simulink model "NeuroControl_Loudspeaker_offline2"  (R2016a)
settings: Solver=ode5  StartTime=0.0  StopTime=0.1  FixedStep=1/fs  RelTol=1e-3
values from neighbouring files (symbols this model uses):
  AaLinear = [0,1,0,0; -(K)/Md,-Rmd/Md,0,A/Md; 0,0,0,1; 0,-A/(L0+Ld),-(1/Cd)/(L0+Ld),-(Re0+Red)/(L0+Ld)]    [NeuroControl_loudspeaker.m]    (also in NeuroControl_loudspeaker2.m; NeuroControl_loudspeaker_LinearPlusNN.m; NeuroControl_loudspeaker_MoreLikeMachineLearning.m; NeuroControl_loudspeaker_MoreLikeMachineLearning_deep.m)
  Anlr = zeros(4,4)    [NeuroControl_loudspeaker.m]    (also in NeuroControl_loudspeaker2.m; NeuroControl_loudspeaker_LinearPlusNN.m; NeuroControl_loudspeaker_MoreLikeMachineLearning.m; NeuroControl_loudspeaker_MoreLikeMachineLearning_deep.m)
  Anlr2 = zeros(4,4)    [NeuroControl_loudspeaker.m]    (also in NeuroControl_loudspeaker2.m; NeuroControl_loudspeaker_LinearPlusNN.m; NeuroControl_loudspeaker_MoreLikeMachineLearning.m; NeuroControl_loudspeaker_MoreLikeMachineLearning_deep.m)
  Anlr3 = zeros(4,4)    [NeuroControl_loudspeaker.m]    (also in NeuroControl_loudspeaker2.m; NeuroControl_loudspeaker_LinearPlusNN.m; NeuroControl_loudspeaker_MoreLikeMachineLearning.m; NeuroControl_loudspeaker_MoreLikeMachineLearning_deep.m)
  Atemp = A    (= 5.62)    [NeuroControl_loudspeaker.m]    (also in NeuroControl_loudspeaker2.m; NeuroControl_loudspeaker_LinearPlusNN.m; NeuroControl_loudspeaker_MoreLikeMachineLearning.m; NeuroControl_loudspeaker_MoreLikeMachineLearning_deep.m)
  Ba = [0,0,0,1/(L0+Ld)]'    [NeuroControl_loudspeaker.m]    (also in NeuroControl_loudspeaker2.m; NeuroControl_loudspeaker_LinearPlusNN.m; NeuroControl_loudspeaker_MoreLikeMachineLearning.m; NeuroControl_loudspeaker_MoreLikeMachineLearning_deep.m)
  fInput = 60    [NeuroControl_loudspeaker.m]    (also in NeuroControl_loudspeaker2.m; NeuroControl_loudspeaker_LinearPlusNN.m; NeuroControl_loudspeaker_MoreLikeMachineLearning.m; NeuroControl_loudspeaker_MoreLikeMachineLearning_deep.m)
  fs = fs/downrate    (= 48000)    [NeuroControl_loudspeaker.m]    (also in NeuroControl_loudspeaker2.m; NeuroControl_loudspeaker_LinearPlusNN.m; NeuroControl_loudspeaker_MoreLikeMachineLearning.m; NeuroControl_loudspeaker_MoreLikeMachineLearning_deep.m)
  fsSim = 48000    [NeuroControl_loudspeaker.m]    (also in NeuroControl_loudspeaker2.m; NeuroControl_loudspeaker_LinearPlusNN.m; NeuroControl_loudspeaker_MoreLikeMachineLearning.m; NeuroControl_loudspeaker_MoreLikeMachineLearning_deep.m)
  G = Gt'    [NeuroControl_loudspeaker.m]    (also in NeuroControl_loudspeaker2.m; NeuroControl_loudspeaker_LinearPlusNN.m; NeuroControl_loudspeaker_MoreLikeMachineLearning.m; NeuroControl_loudspeaker_MoreLikeMachineLearning_deep.m)
  gain = 1/zpkerasys(1,1).k    [NeuroControl_loudspeaker.m]    (also in NeuroControl_loudspeaker2.m; NeuroControl_loudspeaker_LinearPlusNN.m; NeuroControl_loudspeaker_MoreLikeMachineLearning.m; NeuroControl_loudspeaker_MoreLikeMachineLearning_deep.m)
  InputGain = 1    [NeuroControl_loudspeaker.m]    (also in NeuroControl_loudspeaker2.m; NeuroControl_loudspeaker_LinearPlusNN.m; NeuroControl_loudspeaker_MoreLikeMachineLearning.m; NeuroControl_loudspeaker_MoreLikeMachineLearning_deep.m)
  inputGainForPushingNonlinearity = 5    [NeuroControl_loudspeaker.m]    (also in NeuroControl_loudspeaker2.m; NeuroControl_loudspeaker_LinearPlusNN.m = 10; NeuroControl_loudspeaker_MoreLikeMachineLearning.m = 10; NeuroControl_loudspeaker_MoreLikeMachineLearning_deep.m = 10)
  inverseFilterGainCompensation = 1/0.0054    (= 185.185185185)    [NeuroControl_loudspeaker.m]    (also in NeuroControl_loudspeaker2.m; NeuroControl_loudspeaker_LinearPlusNN.m; NeuroControl_loudspeaker_MoreLikeMachineLearning.m; NeuroControl_loudspeaker_MoreLikeMachineLearning_deep.m)
  K = Kd    (= 4538)    [NeuroControl_loudspeaker.m]    (also in NeuroControl_loudspeaker2.m; NeuroControl_loudspeaker_LinearPlusNN.m; NeuroControl_loudspeaker_MoreLikeMachineLearning.m; NeuroControl_loudspeaker_MoreLikeMachineLearning_deep.m)
  noise = 0    [NeuroControl_loudspeaker.m]    (also in NeuroControl_loudspeaker2.m; NeuroControl_loudspeaker_LinearPlusNN.m; NeuroControl_loudspeaker_MoreLikeMachineLearning.m; NeuroControl_loudspeaker_MoreLikeMachineLearning_deep.m)
  ObserverNorm = 1    [NeuroControl_loudspeaker.m]    (also in NeuroControl_loudspeaker2.m; NeuroControl_loudspeaker_LinearPlusNN.m; NeuroControl_loudspeaker_MoreLikeMachineLearning.m; NeuroControl_loudspeaker_MoreLikeMachineLearning_deep.m)
  pole = z_svd    [NeuroControl_loudspeaker.m]    (also in NeuroControl_loudspeaker2.m; NeuroControl_loudspeaker_LinearPlusNN.m; NeuroControl_loudspeaker_MoreLikeMachineLearning.m; NeuroControl_loudspeaker_MoreLikeMachineLearning_deep.m)
  Rmd = 2.34    [NeuroControl_loudspeaker.m]    (also in NeuroControl_loudspeaker2.m; NeuroControl_loudspeaker_LinearPlusNN.m; NeuroControl_loudspeaker_MoreLikeMachineLearning.m; NeuroControl_loudspeaker_MoreLikeMachineLearning_deep.m)
  SignalChange = temp    (= 0)    [NeuroControl_loudspeaker.m]    (also in NeuroControl_loudspeaker2.m; NeuroControl_loudspeaker_LinearPlusNN.m; NeuroControl_loudspeaker_MoreLikeMachineLearning.m; NeuroControl_loudspeaker_MoreLikeMachineLearning_deep.m)
  sys_era_c = d2c(sys_era,'zoh')    [NeuroControl_loudspeaker.m]    (also in NeuroControl_loudspeaker2.m; NeuroControl_loudspeaker_LinearPlusNN.m; NeuroControl_loudspeaker_MoreLikeMachineLearning.m; NeuroControl_loudspeaker_MoreLikeMachineLearning_deep.m)
  zero = zpkerasys(1,1).p{1,1}    [NeuroControl_loudspeaker.m]    (also in NeuroControl_loudspeaker2.m; NeuroControl_loudspeaker_LinearPlusNN.m; NeuroControl_loudspeaker_MoreLikeMachineLearning.m; NeuroControl_loudspeaker_MoreLikeMachineLearning_deep.m)
undefined symbols (not defined in the file or in its folder): a, b
libraries: simulink x1
settings Model: Creator=kadowaki  LastModifiedBy=kadowaki
settings DataIOCC: InspectSignalLogs=on

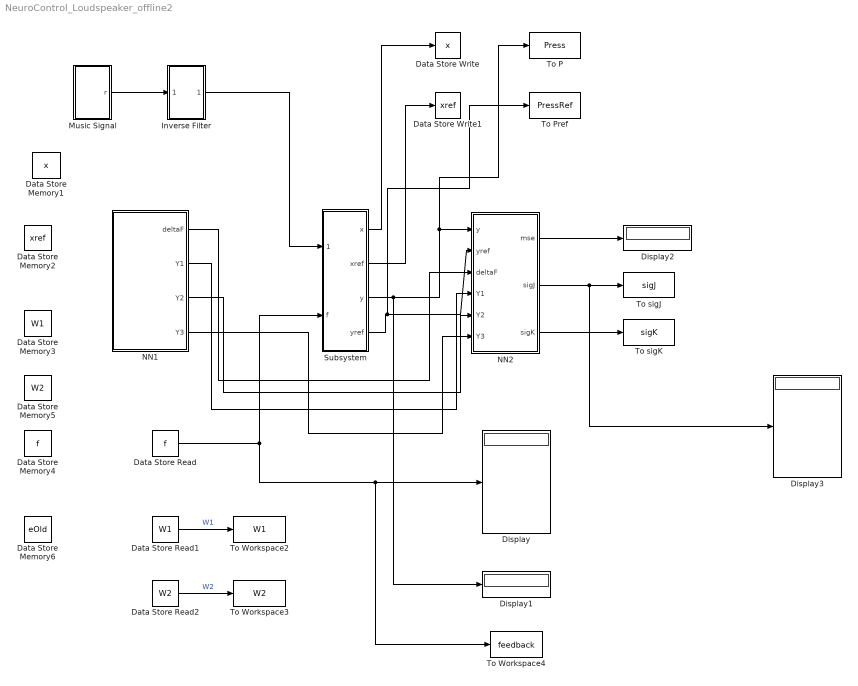
== system NeuroControl_Loudspeaker_offline2 ==
  Data Store Memory1 : DataStoreMemory  DataStoreName=x  ReadBeforeWriteMsg=warning  WriteAfterWriteMsg=warning  WriteAfterReadMsg=warning  InitialValue=zeros(6,1)  ShowAdditionalParam=off  OutDataTypeStr=double
  Data Store Memory2 : DataStoreMemory  DataStoreName=xref  ReadBeforeWriteMsg=warning  WriteAfterWriteMsg=warning  WriteAfterReadMsg=warning  InitialValue=zeros(6,1)  ShowAdditionalParam=off  OutDataTypeStr=double
  Data Store Memory3 : DataStoreMemory  DataStoreName=W1  ReadBeforeWriteMsg=warning  WriteAfterWriteMsg=warning  WriteAfterReadMsg=warning  InitialValue=W1initial  ShowAdditionalParam=off  OutDataTypeStr=double
  Data Store Memory4 : DataStoreMemory  DataStoreName=f  ReadBeforeWriteMsg=warning  WriteAfterWriteMsg=warning  WriteAfterReadMsg=warning  InitialValue=zeros(6,1)  ShowAdditionalParam=off  OutDataTypeStr=double
  Data Store Memory5 : DataStoreMemory  DataStoreName=W2  ReadBeforeWriteMsg=warning  WriteAfterWriteMsg=warning  WriteAfterReadMsg=warning  InitialValue=W2initial  ShowAdditionalParam=off  OutDataTypeStr=double
  Data Store Memory6 : DataStoreMemory  DataStoreName=eOld  ReadBeforeWriteMsg=warning  WriteAfterWriteMsg=warning  WriteAfterReadMsg=warning  ShowAdditionalParam=off  OutDataTypeStr=double
  Data Store Read : DataStoreRead  DataStoreName=f
  Data Store Read1 : DataStoreRead  DataStoreName=W1
  Data Store Read2 : DataStoreRead  DataStoreName=W2
  Data Store Write : DataStoreWrite  DataStoreName=x
  Data Store Write1 : DataStoreWrite  DataStoreName=xref
  Display{,1..3} (4 alike) : Display
  Inverse Filter : Subsystem
  Music Signal : Subsystem
  NN1 : MATLAB Function  TreatAsAtomicUnit=on
      settings: MinAlgLoopOccurrences=on
  NN2 : MATLAB Function  TreatAsAtomicUnit=on
      settings: MinAlgLoopOccurrences=on
  Subsystem : Subsystem
  To P : ToWorkspace  VariableName=Press  SaveFormat=Timeseries  SampleTime=-1
  "To Pref " : ToWorkspace  VariableName=PressRef  SaveFormat=Timeseries  SampleTime=-1
  To Workspace2 : ToWorkspace  VariableName=W1  SampleTime=-1
  To Workspace3 : ToWorkspace  VariableName=W2  SampleTime=-1
  To Workspace4 : ToWorkspace  VariableName=feedback  SampleTime=-1
  To sigJ : ToWorkspace  VariableName=sigJ  SampleTime=-1
  To sigK : ToWorkspace  VariableName=sigK  SampleTime=-1
  wires:
  Subsystem/2(xref) -> Data Store Write1/1
  Subsystem/1(x) -> Data Store Write/1
  Inverse Filter/1(Out1) -> Subsystem/1(music)
  Data Store Read/1 -> To Workspace4/1, Display/1, Subsystem/2(f)
  NN1/1(deltaF) -> NN2/3(deltaF)
  Subsystem/3(y) -> NN2/1(y), To P/1, Display1/1
  Subsystem/4(yref) -> "To Pref "/1, NN2/2(yref)
  NN1/2(Y1) -> NN2/4(Y1)
  NN1/3(Y2) -> NN2/5(Y2)
  Music Signal/1(r) -> Inverse Filter/1(In1)
  NN2/1(mse) -> Display2/1
  NN1/4(Y3) -> NN2/6(Y3)
  Data Store Read1/1 -> To Workspace2/1  "W1"
  Data Store Read2/1 -> To Workspace3/1  "W2"
  NN2/2(sigJ) -> Display3/1, To sigJ/1
  NN2/3(sigK) -> To sigK/1

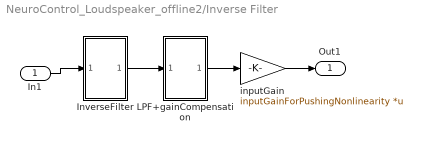
== system NeuroControl_Loudspeaker_offline2/Inverse Filter ==
  In1 : Inport
  InverseFilter : Subsystem
  LPF+gainCompensation : Subsystem
  inputGain : Gain  Gain=inputGainForPushingNonlinearity  Multiplication=Matrix(K*u)
  Out1 : Outport
  wires:
  In1/1 -> InverseFilter/1(In1)
  InverseFilter/1(Out1) -> LPF+gainCompensation/1(In1)
  LPF+gainCompensation/1(Out1) -> inputGain/1
  inputGain/1 -> Out1/1

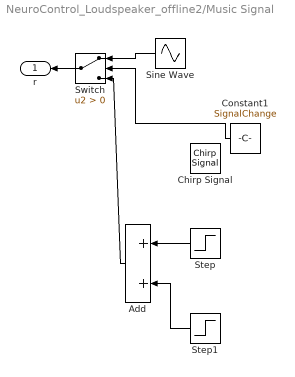
== system NeuroControl_Loudspeaker_offline2/Music Signal ==
  Add : Sum
  Chirp Signal : simulink/Sources/Chirp Signal  f1=0.1  T=2  f2=fs/2
  Constant1 : Constant  Value=SignalChange
  Sine Wave : Sin  Amplitude=InputGain  Frequency=2*pi*fInput  SampleTime=[0,0]
  Step : Step  Time=0  After=InputGain  SampleTime=[0,0]
  Step1 : Step  Time=1/fsSim  After=-InputGain  SampleTime=[0,0]
  Switch : Switch  Criteria=u2 > Threshold
  r : Outport
  wires:
  Switch/1 -> r/1
  Constant1/1 -> Switch/2
  Sine Wave/1 -> Switch/1
  Step/1 -> Add/1
  Add/1 -> Switch/3
  Step1/1 -> Add/2

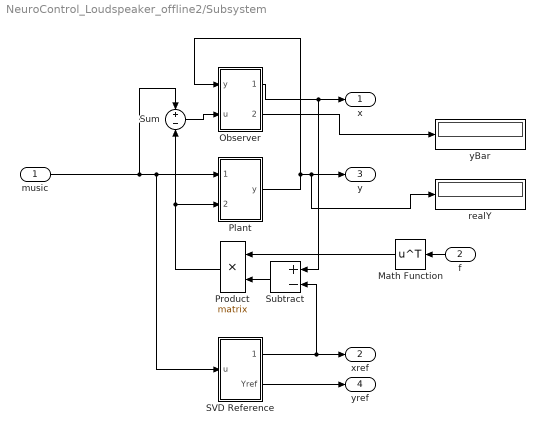
== system NeuroControl_Loudspeaker_offline2/Subsystem ==
  music : Inport
  f : Inport  Port=2
  Math Function : Math  Operator=transpose  SaturateOnIntegerOverflow=on
  Observer : Subsystem
  Plant : Subsystem
  Product : Product  Multiplication=Matrix(*)
  SVD Reference : Subsystem
  Subtract : Sum  Inputs=+-
  Sum : Sum  Inputs=+-
  realY : Display
  yBar : Display
  x : Outport
  xref : Outport  Port=2
  y : Outport  Port=3
  yref : Outport  Port=4
  wires:
  Plant/1(y) -> realY/1, y/1, Observer/1(y)
  music/1 -> Sum/1, SVD Reference/1(u), Plant/1(music)
  SVD Reference/1(Xref) -> Subtract/2, xref/1
  Observer/1(xBar) -> Subtract/1, x/1
  SVD Reference/2(Yref) -> yref/1
  f/1 -> Math Function/1
  Math Function/1 -> Product/1
  Subtract/1 -> Product/2
  Observer/2(yBar) -> yBar/1
  Product/1 -> Sum/2, Plant/2(control)
  Sum/1 -> Observer/2(u)

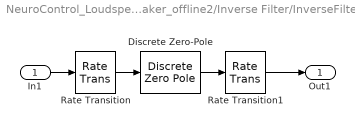
== system NeuroControl_Loudspeaker_offline2/Inverse Filter/InverseFilter ==
  In1 : Inport
  Discrete Zero-Pole : DiscreteZeroPole  Zeros=zero  Poles=pole  Gain=gain  SampleTime=1/fs
  Rate Transition : RateTransition
  Rate Transition1 : RateTransition
  Out1 : Outport
  wires:
  Rate Transition/1 -> Discrete Zero-Pole/1
  Discrete Zero-Pole/1 -> Rate Transition1/1
  In1/1 -> Rate Transition/1
  Rate Transition1/1 -> Out1/1

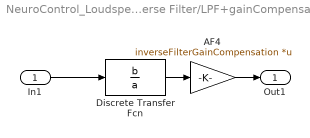
== system NeuroControl_Loudspeaker_offline2/Inverse Filter/LPF+gainCompensation ==
  In1 : Inport
  AF4 : Gain  Gain=inverseFilterGainCompensation  Multiplication=Matrix(K*u)
  Discrete Transfer Fcn : DiscreteTransferFcn  Numerator=b  Denominator=a
  Out1 : Outport
  wires:
  Discrete Transfer Fcn/1 -> AF4/1
  AF4/1 -> Out1/1
  In1/1 -> Discrete Transfer Fcn/1

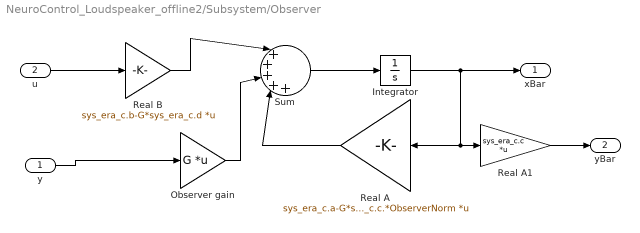
== system NeuroControl_Loudspeaker_offline2/Subsystem/Observer ==
  y : Inport
  u : Inport  Port=2
  Integrator : Integrator
  Observer gain : Gain  Gain=G  Multiplication=Matrix(K*u)
  Real A : Gain  Gain=sys_era_c.a-G*sys_era_c.c.*ObserverNorm  Multiplication=Matrix(K*u)
  Real A1 : Gain  Gain=sys_era_c.c  Multiplication=Matrix(K*u)
  Real B : Gain  Gain=sys_era_c.b-G*sys_era_c.d  Multiplication=Matrix(K*u)
  Sum : Sum  Inputs=|+++++
  xBar : Outport
  yBar : Outport  Port=2
  wires:
  Sum/1 -> Integrator/1
  Integrator/1 -> Real A1/1, Real A/1, xBar/1
  Real A/1 -> Sum/4
  u/1 -> Real B/1
  Real B/1 -> Sum/1
  y/1 -> Observer gain/1
  Observer gain/1 -> Sum/3
  Real A1/1 -> yBar/1

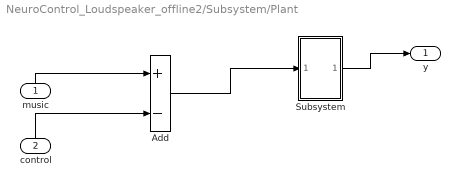
== system NeuroControl_Loudspeaker_offline2/Subsystem/Plant ==
  music : Inport
  control : Inport  Port=2
  Add : Sum  Inputs=+-
  Subsystem : Subsystem  TreatAsAtomicUnit=on
      settings: MinAlgLoopOccurrences=on
  y : Outport
  wires:
  Subsystem/1(Out1) -> y/1
  music/1 -> Add/1
  control/1 -> Add/2
  Add/1 -> Subsystem/1(In2)

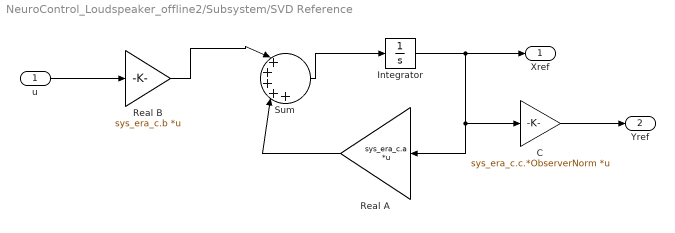
== system NeuroControl_Loudspeaker_offline2/Subsystem/SVD Reference ==
  u : Inport
  C : Gain  Gain=sys_era_c.c.*ObserverNorm  Multiplication=Matrix(K*u)
  Integrator : Integrator
  Real A : Gain  Gain=sys_era_c.a  Multiplication=Matrix(K*u)
  Real B : Gain  Gain=sys_era_c.b  Multiplication=Matrix(K*u)
  Sum : Sum  Inputs=|+++++
  Xref : Outport
  Yref : Outport  Port=2
  wires:
  Sum/1 -> Integrator/1
  Integrator/1 -> Real A/1, C/1, Xref/1
  Real A/1 -> Sum/4
  u/1 -> Real B/1
  Real B/1 -> Sum/1
  C/1 -> Yref/1

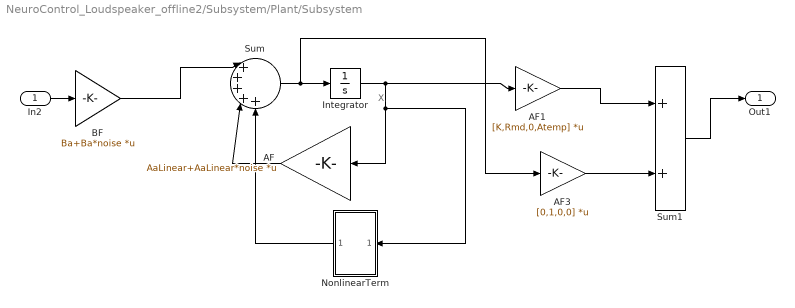
== system NeuroControl_Loudspeaker_offline2/Subsystem/Plant/Subsystem ==
  note: X
  In2 : Inport
  AF : Gain  Gain=AaLinear+AaLinear*noise  Multiplication=Matrix(K*u)
  AF1 : Gain  Gain=[K,Rmd,0,Atemp]  Multiplication=Matrix(K*u)
  AF3 : Gain  Gain=[0,1,0,0]  Multiplication=Matrix(K*u)
  BF : Gain  Gain=Ba+Ba*noise  Multiplication=Matrix(K*u)
  Integrator : Integrator
  NonlinearTerm : Subsystem
  Sum : Sum  Inputs=|+++++
  Sum1 : Sum
  Out1 : Outport
  wires:
  BF/1 -> Sum/1
  Sum/1 -> Integrator/1, AF3/1
  Integrator/1 -> AF/1, NonlinearTerm/1(In1), AF1/1
  AF/1 -> Sum/4
  NonlinearTerm/1(Out2) -> Sum/5
  In2/1 -> BF/1
  AF1/1 -> Sum1/1
  Sum1/1 -> Out1/1
  AF3/1 -> Sum1/2

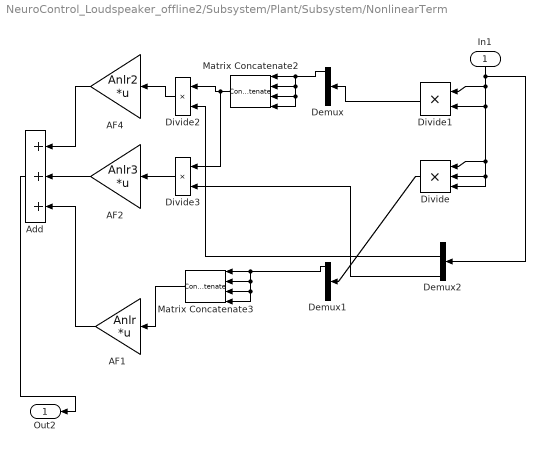
== system NeuroControl_Loudspeaker_offline2/Subsystem/Plant/Subsystem/NonlinearTerm ==
  In1 : Inport
  AF1 : Gain  Gain=Anlr  Multiplication=Matrix(K*u)
  AF2 : Gain  Gain=Anlr3  Multiplication=Matrix(K*u)
  AF4 : Gain  Gain=Anlr2  Multiplication=Matrix(K*u)
  Add : Sum  Inputs=+++
  Demux : Demux  Outputs=[1,1,1,1]
  Demux1 : Demux  Outputs=[1,1,1,1]
  Demux2 : Demux  Outputs=[1,1,1,1]
  Divide : Product  Inputs=***
  Divide1 : Product  Inputs=**
  Divide2 : Product  Inputs=**
  Divide3 : Product  Inputs=**
  Matrix Concatenate2 : Concatenate  NumInputs=4
  Matrix Concatenate3 : Concatenate  NumInputs=4
  Out2 : Outport
  wires:
  Matrix Concatenate3/1 -> AF1/1
  Divide/1 -> Demux1/1
  In1/1 -> Demux2/1, Divide1/2, Divide/2, Divide/3, Divide/1, Divide1/1
  Demux/1 -> Matrix Concatenate2/1, Matrix Concatenate2/2, Matrix Concatenate2/3, Matrix Concatenate2/4
  Demux1/1 -> Matrix Concatenate3/1, Matrix Concatenate3/2, Matrix Concatenate3/3, Matrix Concatenate3/4
  AF2/1 -> Add/2
  AF4/1 -> Add/1
  AF1/1 -> Add/3
  Add/1 -> Out2/1
  Matrix Concatenate2/1 -> Divide2/1, Divide3/1
  Demux2/2 -> Divide2/2
  Divide2/1 -> AF4/1
  Divide3/1 -> AF2/1
  Demux2/4 -> Divide3/2
  Divide1/1 -> Demux/1

== matlab function NeuroControl_Loudspeaker_offline2/NN2 ==
  data: y input; yref input; deltaF input; W1 data_store_memory; W2 data_store_memory; eOld data_store_memory; Y1 input; Y2 input; mse output; Y3 input; sigJ output; sigK output
function [mse,sigJ,sigK]  = fcn(y,yref,deltaF,Y1,Y2,Y3)
%% cost関数をatctual plantの出力YとYrefの差の二乗和の形に書き換える。それにともなってsigKとかも変わる
%%%%%%%%%%%%%%%%%%%%%%%%%%%%%%%%%%%%%%%%%%%%%%%%%%%%%%%%%%%%%%%%%%%%%%%%%%%%%%%%%%%%%%%%%%%%%%%%%%%%%%%%%%%%
%%

%#codegen
%配列は縦で入れる
%PRMLの5.3.2
%隠れ層はtanh,出力層は線形の活性化関数
% Input:
%   x: state vector of a plant
%   xref: reference state vector
%   h: 隠れ層のニューロン数
% Ouput:
%   du: input to compensate plant nonlinearity
%   mse: mean square error
%12input-1outputのニューラルネット
%フィードバックの機構いる？ニューラルネットだけではだめなのか。
%実装に際しては，1サンプル中にニューラルネットの計算が終わるのかという問題はある。

%過去のグローバル変数定義
global W1
global W2
%yOldの初期条件を設定するためだけにグローバル変数導入。きっともっといい方法がある。
global eOld
eta = 0.00000000000000001;

%コスト関数

%ヤコビアンを求める
deltaY = y - yref - eOld;
sign = deltaY*deltaF;
%signが負のjacobi要素は-1に他は+1
jacobi = sign>0;
jacobi = jacobi - (jacobi == 0);
%jacobi = jacobi*(-1);

%%
%出力層ユニットに対するsigmaK
%tanh
sigK = (y - yref)*jacobi.*(1-Y3.^2);
% %linear
%sigK = (y - yref)*jacobi;
%     backward
E = y - yref;
mse = mean(dot(E(:),E(:)));

%中間層
%tanh
%sigJ = (1-Y2.^2).*(W2*sigK);
%sigmoid
sigJ = Y2.*(1-Y2).*(W2*sigK);

W1 = W1-eta*(Y1*sigJ');
W2 = W2-eta*(Y2*sigK');

eOld = y - yref;

== matlab function NeuroControl_Loudspeaker_offline2/NN1 ==
  data: xref data_store_memory; f data_store_memory; deltaF output; Y1 output; Y2 output; W1 data_store_memory; W2 data_store_memory; x data_store_memory; Y3 output
function [deltaF,Y1,Y2,Y3]  = fcn
%% cost関数をatctual plantの出力YとYrefの差の二乗和の形に書き換える。それにともなってsigKとかも変わる
%%%%%%%%%%%%%%%%%%%%%%%%%%%%%%%%%%%%%%%%%%%%%%%%%%%%%%%%%%%%%%%%%%%%%%%%%%%%%%%%%%%%%%%%%%%%%%%%%%%%%%%%%%%%
%%

%#codegen
%配列は縦で入れる
%ニューラルネットの順伝播で出力求める。
%出力はフィードバックゲインf

%グローバル変数定義
global x
global xref
global f
global W1
global W2


%x,xrefは縦ベクトルでなければならない
Y1 = [1;x;xref];

%forward
%中間層出力
%活性化関数定義
Y2 = tanh(W1'*Y1)/10;
%Y2 = sigmoid(W1'*Y1);

%出力層出力
%linear
%Y3 = W2'*Y2;
%tanh
Y3 = tanh(W2'*Y2)/10;

%ユニット出力（今はフィードバックゲイン）の差分
deltaF = Y3 - f;
f = Y3;
